simulink model "DiscreteIntegrator_TestGen9"  (R2017b)
settings: Solver=FixedStepDiscrete  StartTime=0.0  StopTime=10.0  RelTol=1e-3
undefined symbols (not defined in the file): Block_TestLib, DiscIntNeverNeededParam, enable
settings Model: Creator=hbourbou  LastModifiedBy=hbourbou
settings DebuggingCC: ParameterOverflowMsg=none

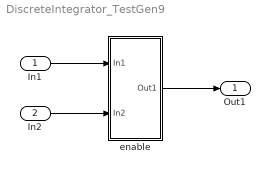
== system DiscreteIntegrator_TestGen9 ==
  In1 : Inport
  In2 : Inport  Port=2
  enable : Subsystem  AncestorBlock=Block_TestLib/enable
  Out1 : Outport
  wires:
  In1/1 -> enable/1(In1)
  In2/1 -> enable/2(In2)
  enable/1(Out1) -> Out1/1

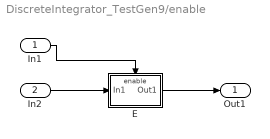
== system DiscreteIntegrator_TestGen9/enable ==
  In1 : Inport  OutDataTypeStr=boolean
  In2 : Inport  Port=2
  E : Subsystem  TreatAsAtomicUnit=on
  Out1 : Outport
  wires:
  In1/1 -> E/Enable
  In2/1 -> E/1(In1)
  E/1(Out1) -> Out1/1

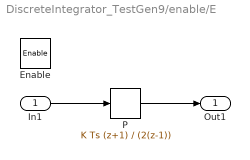
== system DiscreteIntegrator_TestGen9/enable/E ==
  In1 : Inport  OutDataTypeStr=double  PortDimensions=[2,3]
  Enable : EnablePort
  P : DiscreteIntegrator  IntegratorMethod=Integration: Trapezoidal  InitialCondition=7  InitialConditionSetting=State (most efficient)  SampleTime=-1  OutDataTypeStr=double  RndMeth=Convergent  UpperSaturationLimit=100  LowerSaturationLimit=5  ICPrevOutput=DiscIntNeverNeededParam  ICPrevScaledInput=DiscIntNeverNeededParam
  Out1 : Outport
  wires:
  In1/1 -> P/1
  P/1 -> Out1/1
